simulink model "interpolation_nD_TestGen36"  (R2017b)
settings: Solver=FixedStepDiscrete  StartTime=0.0  StopTime=10.0  RelTol=1e-3
PreLoadFcn:
  |  LUTObj = Simulink.LookupTable;
  |  LUTObj.Table.Value = [74.4364083057892 15.025584654915;57.9460761104725 0.0707958435945909;57.6357055109509 114.836843052068];
  |  LUTObj.Table.DataType = 'auto';
  |  LUTObj.StructTypeInfo.Name = 'myLUTStruct';
  |  LUTObj.BreakpointsSpecification = 'Reference';
  |  LUTObj.Breakpoints{1} = 'myBpSet1';
  | myBpSet1 = Simulink.Breakpoint;
  | myBpSet1.Breakpoints.Value = [1 2 3];
  |  LUTObj.Breakpoints{2} = 'myBpSet2';
  | myBpSet2 = Simulink.Breakpoint;
  | myBpSet2.Breakpoints.Value = [1 2];
settings Model: Creator=ktrinh  LastModifiedBy=ktrinh
settings DebuggingCC: ParameterOverflowMsg=none

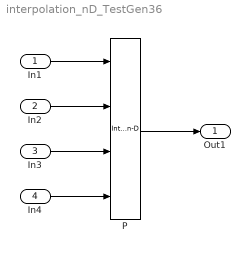
== system interpolation_nD_TestGen36 ==
  In1 : Inport  OutMin=0  OutMax=3  PortDimensions=1
  In2 : Inport  Port=2  OutMin=-0.5  OutMax=1.5
  In3 : Inport  Port=3  OutMin=0  OutMax=2
  In4 : Inport  Port=4  OutMin=-0.5  OutMax=1.5
  P : Interpolation_n-D  Table=[74.4364083057892 15.025584654915;57.9460761104725 0.0707958435945909;57.6357055109509 114.836843052068]  TableSpecification=Lookup table object  LookupTableObject=LUTObj  InternalRulePriority=Speed  RndMeth=Convergent
  Out1 : Outport
  wires:
  In1/1 -> P/1
  In2/1 -> P/2
  In3/1 -> P/3
  In4/1 -> P/4
  P/1 -> Out1/1
